simulink model "phan1_bai3a"  (R2019a)
settings: Solver=VariableStepAuto  StartTime=0.0  StopTime=60  RelTol=1e-3
values from neighbouring files (symbols this model uses):
  Tstep = 0.01    [phan1_bai2a_kieu1_test.m]    (also in phan1_bai2a_kieu2_test.m; phan1_bai2b_kieu1_test.m; phan1_bai2b_kieu2_test.m; phan1_bai2c_kieu1_test.m)
libraries: simulink x1
settings Model: Creator=inhuo  LastModifiedBy=inhuo

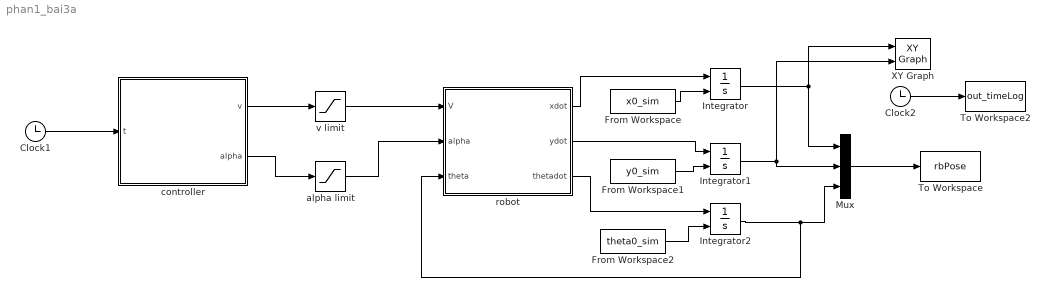
== system phan1_bai3a ==
  Clock1 : Clock
  Clock2 : Clock
  From Workspace : FromWorkspace  VariableName=x0_sim  SampleTime=0  OutputAfterFinalValue=Holding final value
  From Workspace1 : FromWorkspace  VariableName=y0_sim  SampleTime=0  OutputAfterFinalValue=Holding final value
  From Workspace2 : FromWorkspace  VariableName=theta0_sim  SampleTime=0  OutputAfterFinalValue=Holding final value
  Integrator : Integrator  InitialConditionSource=external
  Integrator1 : Integrator  InitialConditionSource=external
  Integrator2 : Integrator  InitialConditionSource=external
  Mux : Mux  Inputs=3
  To Workspace : ToWorkspace  VariableName=rbPose  SampleTime=Tstep
  To Workspace2 : ToWorkspace  VariableName=out_timeLog  SampleTime=-1
      settings: Save2DSignal=2-D array (concatenate along first dimension)
  XY Graph : simulink/Sinks/XY Graph  xmin=-1  xmax=25  ymin=-10  ymax=1  st=-1
  alpha limit : Saturate  UpperLimit=pi/4  LowerLimit=-pi/4
  controller : MATLAB Function  TreatAsAtomicUnit=on
  "robot " : MATLAB Function  TreatAsAtomicUnit=on
  "v limit " : Saturate  UpperLimit=1.77  LowerLimit=-1.77
  wires:
  Clock1/1 -> controller/1(t)
  controller/1(v) -> "v limit "/1
  "v limit "/1 -> "robot "/1(V)
  controller/2(alpha) -> alpha limit/1
  alpha limit/1 -> "robot "/2(alpha)
  From Workspace1/1 -> Integrator1/2
  From Workspace/1 -> Integrator/2
  From Workspace2/1 -> Integrator2/2
  Mux/1 -> To Workspace/1
  "robot "/1(xdot) -> Integrator/1
  "robot "/2(ydot) -> Integrator1/1
  Clock2/1 -> To Workspace2/1
  "robot "/3(thetadot) -> Integrator2/1
  Integrator1/1 -> Mux/2, XY Graph/2
  Integrator/1 -> Mux/1, XY Graph/1
  Integrator2/1 -> Mux/3, "robot "/3(theta)

== matlab function phan1_bai3a/controller ==
  data: v output; t input; alpha output
function [v, alpha] = fcn(t)
    % Setup Config
    G = 9;
    d = sqrt(2.5 + 0.1*G); % Axial Space
    
    if t < 20
        v = 1;
        alpha = 0;
    elseif (t >= 20) && ( t<= 40)
        v = pi/5;    
        alpha = -atan2(d, 4);
    elseif (t >= 41) && (t <= 61)
        v = 1;
        alpha = 0;
    else
        v = 0;
        alpha = 0;
    end
end

== matlab function phan1_bai3a/robot  ==
  data: V input; xdot output; alpha input; theta input; ydot output; thetadot output
function [xdot , ydot , thetadot]= fcn(V,alpha,theta)
    d = sqrt(2.5 + 0.1*9); 

    % Kinematic Equations
    xdot = V * cos(theta);
    ydot = V * sin(theta);
    thetadot = V * tan(alpha)/d;
end

% case 1 
%      xdot = V*cos(alpha)*cos(theta);
%      ydot = V*cos(alpha)*sin(theta);
%      thetadot =V*sin(alpha)/d;

% case 2
% xdot = V*cos(theta);
% ydot = V*sin(theta);
% thetadot =V*tan(alpha)/d;
